simulink model "CodeGen"  (R2024b)
settings: Solver=FixedStepDiscrete  StartTime=0  StopTime=511  FixedStep=1/128  RelTol=1e-3
InitFcn:
  | load('ECG_Data_split.mat')
  | ecg_stream = timetable(testData','TimeStep',seconds(1/128));
  | classNames=["ARR","CHF","NSR"];
  | classNamesL=["arr","chf","nsr"];
  | path = ['CodeGen','/Subsystem/ECG Preprocessing/LSTM_Version/Resettable Subsystem/Stateful Classify1/'];
  | set_param(path,'InputDataFormats',"{'sequenceinput', 'CT'}");
undefined symbols (not defined in the file): gray
libraries: deeplib x2, dspfeatures x1, pil_lib x1
settings Model: Creator=The MathWorks, Inc.  LastModifiedBy=resjoehr
settings SolverCC: AlgebraicLoopSolver=TrustRegion
settings OptimizationCC: DefaultParameterBehavior=Inlined  EnhancedBackFolding=on  PassReuseOutputArgsAs=Individual arguments  ZeroExternalMemoryAtStartup=off  ZeroInternalMemoryAtStartup=off  InitFltsAndDblsToZero=on  MaxStackSize=200000  OptimizeBlockOrder=speed  DifferentSizesBufferReuse=on  OptimizationCustomize=off  EfficientTunableParamExpr=on
settings DebuggingCC: ParameterTunabilityLossMsg=error  UnconnectedInputMsg=warning  UnconnectedOutputMsg=warning  UnconnectedLineMsg=warning
settings HardwareCC: ProdBitPerLong=64  ProdLargestAtomicInteger=LongLong  ProdLargestAtomicFloat=Double  ProdLongLongMode=on  ProdHWDeviceType=ARM Compatible->ARM Cortex-A (64-bit)  TargetLongLongMode=on
settings ModelReferenceCC: EnableRefExpFcnMdlSchedulingChecks=on
settings SFSimCC: SimTargetLang=C++  SimGPUErrorChecks=on
settings RTWCC: Description=Embedded Coder  SystemTargetFile=ert.tlc  HardwareBoard=NVIDIA Jetson  TLCOptions="-aInlineSetEventsForThisBaseRateFcn=TLC_FALSE -aSuppressMultiTaskScheduler=TLC_FALSE  -aRateBasedStepFcn=0"  TemplateMakefile=ert_default_tmf  GenerateReport=on  LaunchReport=on  CreateSILPILBlock=PIL  TargetLang=C++  GenerateGPUCode=CUDA  GenerateCodeMetricsReport=on  GPUComputeCapability=3.5  DLArmComputeVersion=19.05
settings CodeAppCC: ForceParamTrailComments=on  IgnoreCustomStorageClasses=off  OperatorAnnotations=on  SimulinkDataObjDesc=on  SFDataObjDesc=on  InsertBlockDesc=on
settings ERTTargetCC: CodeInterfacePackaging=C++ class  SupportVariableSizeSignals=on  RootIOFormat=Structure reference  DynamicArrayContainerType=coder::array

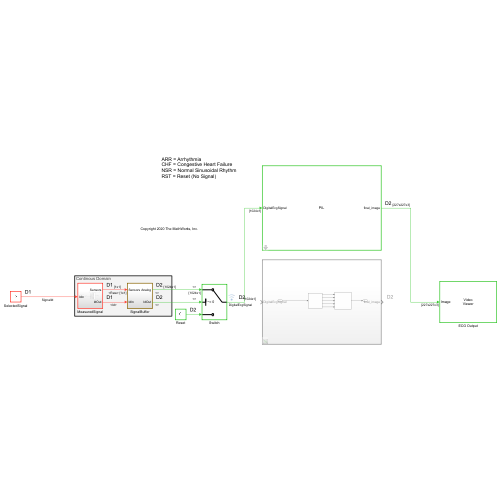
[thumbnail: Simulink's stored preview of the top-level diagram]
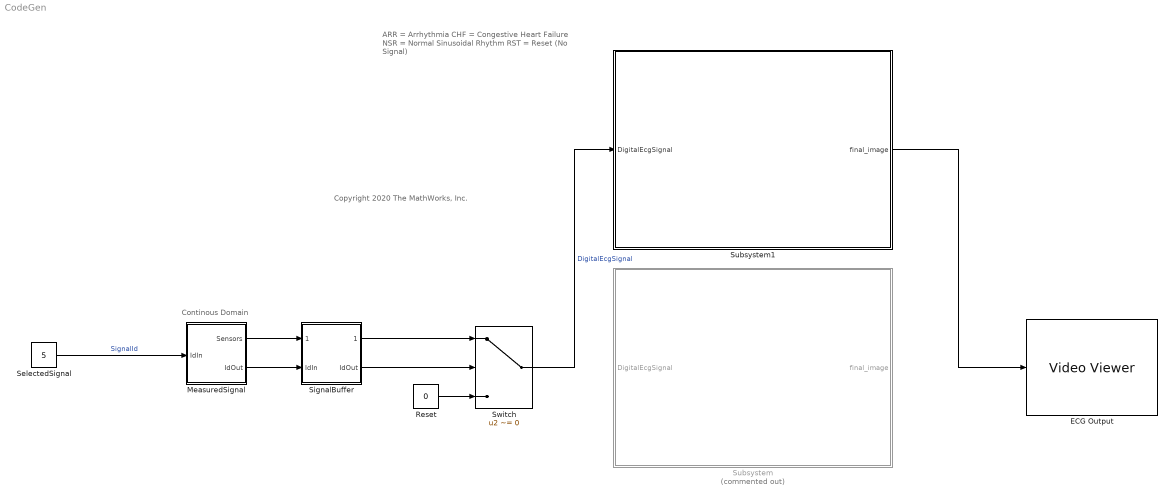
== system CodeGen ==
  note: Copyright 2020 The MathWorks, Inc.
  note: ARR = Arrhythmia
      | CHF = Congestive Heart Failure
      | NSR = Normal Sinusoidal Rhythm
      | RST = Reset (No Signal)
  note: Continous Domain
  ECG Output : VideoViewer  colormapValue=gray(256)  FigPos=[-1729 1066.66666666667 1030.66666666667 710]
  MeasuredSignal : Subsystem  VariantControl=testMixed
  Reset : Constant  Value=0  SampleTime=-1
  SelectedSignal : Constant  Value=5  SampleTime=-1
  SignalBuffer : Subsystem
  Subsystem : Subsystem  Commented=on  TreatAsAtomicUnit=on
  Subsystem1 : Subsystem  DialogController=pil_create_dialog  LoadFcn=|
      | try
      |    if ~strcmp(rtw.pil.getPILVersion, '24.2 (R2024b)_15')
      |       set_param(gcb, 'DialogController', '');
      |       set_param(gcb, 'DialogControllerArgs', '');
      |    end
      | catch e
      |       set_param(gcb, 'DialogController', '');
      |       set_param(gcb, 'DialogControllerArgs', '');
      | end
      mask help: PIL:pil:XILBlockMaskDesc
      mask Display: disp('PIL');
  Switch : Switch  Criteria=u2 ~= 0  OutDataTypeStr=Inherit: Inherit via back propagation  SaturateOnIntegerOverflow=off  InputSameDT=off
  wires:
  SignalBuffer/1(Analog) -> Switch/1
  SelectedSignal/1 -> MeasuredSignal/1(IdIn)  "SignalId"
  MeasuredSignal/1(Sensors) -> SignalBuffer/1(Sensors)
  SignalBuffer/2(IdOut) -> Switch/2
  MeasuredSignal/2(IdOut) -> SignalBuffer/2(IdIn)
  Reset/1 -> Switch/3
  Switch/1 -> Subsystem1/1(DigitalEcgSignal)  "DigitalEcgSignal"
  Subsystem1/1(final_image) -> ECG Output/1

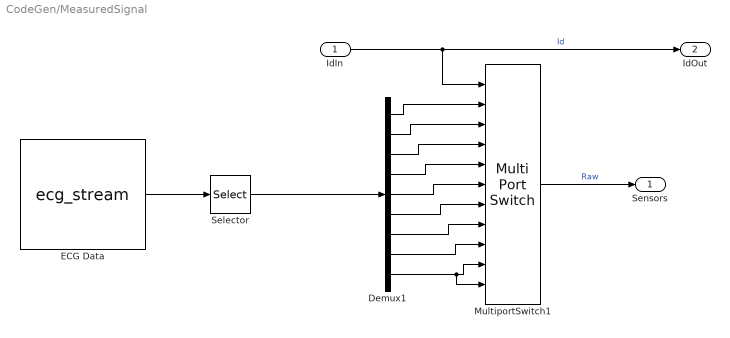
== system CodeGen/MeasuredSignal ==
  IdIn : Inport
  Demux1 : Demux  Outputs=9
  ECG Data : FromWorkspace  VariableName=ecg_stream  SampleTime=1/128
  MultiportSwitch1 : MultiPortSwitch  Inputs=9  DataPortForDefault=Additional data port  DiagnosticForDefault=None  SaturateOnIntegerOverflow=off  InputSameDT=off
  Selector : Selector  InputPortWidth=49  IndexOptions=Index vector (dialog)  Indices=[3 12 27 31 36 38 43 48 49]  OutputSizes=1
  Sensors : Outport
  IdOut : Outport  Port=2
  wires:
  IdIn/1 -> MultiportSwitch1/1, IdOut/1  "Id"
  Demux1/8 -> MultiportSwitch1/9
  Selector/1 -> Demux1/1
  Demux1/9 -> MultiportSwitch1/11, MultiportSwitch1/10
  Demux1/7 -> MultiportSwitch1/8
  Demux1/4 -> MultiportSwitch1/5
  Demux1/5 -> MultiportSwitch1/6
  MultiportSwitch1/1 -> Sensors/1  "Raw"
  ECG Data/1 -> Selector/1
  Demux1/6 -> MultiportSwitch1/7
  Demux1/1 -> MultiportSwitch1/2
  Demux1/3 -> MultiportSwitch1/4
  Demux1/2 -> MultiportSwitch1/3

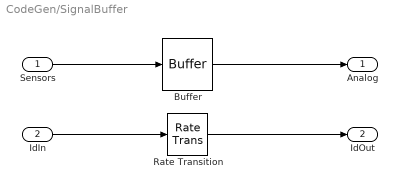
== system CodeGen/SignalBuffer ==
  Sensors : Inport
  IdIn : Inport  Port=2
  Buffer : Buffer  N=1024  V=512  OutputFrames=off
  Rate Transition : RateTransition  OutPortSampleTime=4
  Analog : Outport
  IdOut : Outport  Port=2
  wires:
  IdIn/1 -> Rate Transition/1
  Sensors/1 -> Buffer/1
  Buffer/1 -> Analog/1
  Rate Transition/1 -> IdOut/1

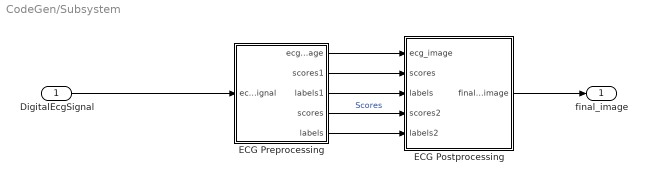
== system CodeGen/Subsystem ==
  DigitalEcgSignal : Inport
  ECG Postprocessing : MATLAB Function  TreatAsAtomicUnit=on
  ECG Preprocessing : Subsystem  TreatAsAtomicUnit=on
  final_image : Outport
  wires:
  ECG Preprocessing/4(scores) -> ECG Postprocessing/4(scores2)  "Scores"
  ECG Preprocessing/5(labels) -> ECG Postprocessing/5(labels2)
  ECG Preprocessing/1(ecg_image) -> ECG Postprocessing/1(ecg_image)
  DigitalEcgSignal/1 -> ECG Preprocessing/1(ecg_signal)
  ECG Postprocessing/1(final_image) -> final_image/1
  ECG Preprocessing/3(labels1) -> ECG Postprocessing/3(labels)
  ECG Preprocessing/2(scores1) -> ECG Postprocessing/2(scores)

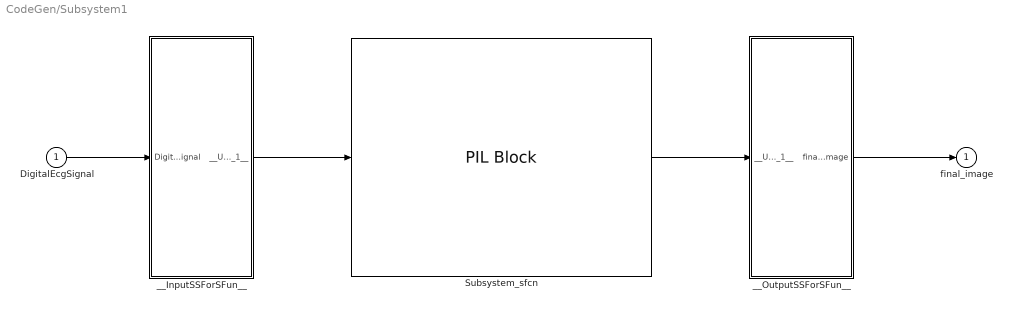
== system CodeGen/Subsystem1 ==
  DigitalEcgSignal : Inport
  Subsystem_sfcn : pil_lib/PIL Block  SimulationMode=PIL  IsTopModelPIL=off  CodeDir=Subsystem_ert_rtw  AnchorDir=C:\MATLAB\Content\D1_Artificial_Intelligence\M3_Workshops\AdaptedMaterial\AMLD_2025_final\Ch4_Deployment  ConfigName=NVIDIA Jetson  XrelIsTopModelCode=on  XrelIsReusable=off  XrelDWorkNames={}  XrelDWorkTypes={}  XrelModelArgVals={}  XrelOrderedParamNames={}  XRelNonFiniteStyle=NONFINITE_UNUSED
  __InputSSForSFun__ : Subsystem
  __OutputSSForSFun__ : Subsystem
  final_image : Outport
  wires:
  DigitalEcgSignal/1 -> __InputSSForSFun__/1(DigitalEcgSignal)
  __InputSSForSFun__/1(__UniqueOutportName__1__) -> Subsystem_sfcn/1
  Subsystem_sfcn/1 -> __OutputSSForSFun__/1(__UniqueInportName__1__)
  __OutputSSForSFun__/1(final_image) -> final_image/1

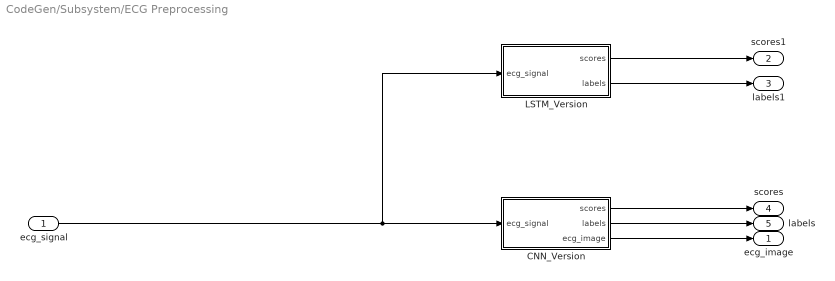
== system CodeGen/Subsystem/ECG Preprocessing ==
  ecg_signal : Inport
  CNN_Version : Subsystem  TreatAsAtomicUnit=on  VariantControl=false
      settings: RTWSystemCode=Nonreusable function
  LSTM_Version : Subsystem  TreatAsAtomicUnit=on  VariantControl=true
      settings: RTWSystemCode=Nonreusable function
  ecg_image : Outport
  scores1 : Outport  Port=2
  labels1 : Outport  Port=3
  scores : Outport  Port=4
  labels : Outport  Port=5
  wires:
  ecg_signal/1 -> LSTM_Version/1(ecg_signal), CNN_Version/1(ecg_signal)
  CNN_Version/3(ecg_image) -> ecg_image/1
  CNN_Version/2(labels) -> labels/1
  CNN_Version/1(scores) -> scores/1
  LSTM_Version/1(scores) -> scores1/1
  LSTM_Version/2(labels) -> labels1/1

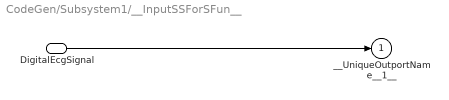
== system CodeGen/Subsystem1/__InputSSForSFun__ ==
  DigitalEcgSignal : Inport
  __UniqueOutportName__1__ : Outport
  wires:
  DigitalEcgSignal/1 -> __UniqueOutportName__1__/1

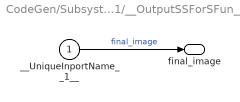
== system CodeGen/Subsystem1/__OutputSSForSFun__ ==
  __UniqueInportName__1__ : Inport
  final_image : Outport
  wires:
  __UniqueInportName__1__/1 -> final_image/1  "final_image"

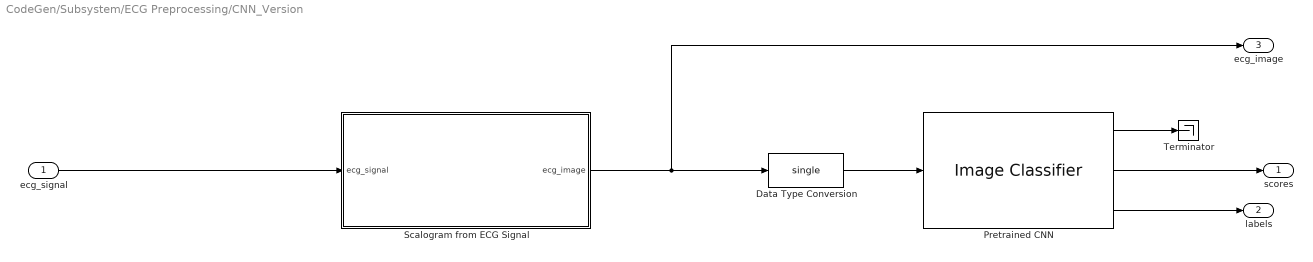
== system CodeGen/Subsystem/ECG Preprocessing/CNN_Version ==
  ecg_signal : Inport
  Data Type Conversion : DataTypeConversion  OutDataTypeStr=single  SaturateOnIntegerOverflow=off  RndMeth=Floor
  "Pretrained CNN " : deeplib/Image Classifier  Network=Network from MAT-file  NetworkFunction=squeezenet  NetworkFilePath=trained_GN.mat  NetworkClassesVariable=classNames  MiniBatchSize=128  ResizeInput=on  Classification=on  Predictions=on  ForceInterpretedSim=off  PredictMode=All probabilities and labels  K=5
  Scalogram from ECG Signal : MATLAB Function  TreatAsAtomicUnit=on
  Terminator : Terminator
  scores : Outport
  labels : Outport  Port=2
  ecg_image : Outport  Port=3
  wires:
  Data Type Conversion/1 -> "Pretrained CNN "/1
  Scalogram from ECG Signal/1(ecg_image) -> ecg_image/1, Data Type Conversion/1
  ecg_signal/1 -> Scalogram from ECG Signal/1(ecg_signal)
  "Pretrained CNN "/1 -> Terminator/1
  "Pretrained CNN "/2 -> scores/1
  "Pretrained CNN "/3 -> labels/1

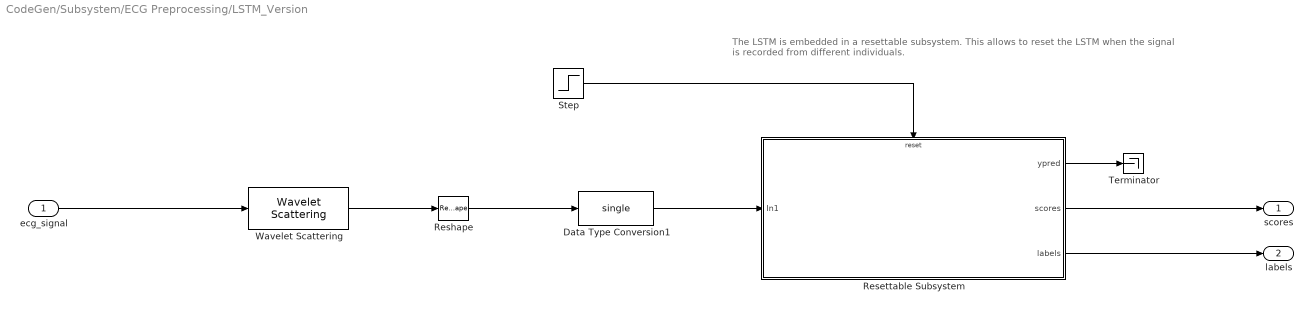
== system CodeGen/Subsystem/ECG Preprocessing/LSTM_Version ==
  note: The LSTM is embedded in a resettable subsystem. This allows to reset the LSTM when the signal is recorded from different individuals.
  ecg_signal : Inport
  Data Type Conversion1 : DataTypeConversion  OutDataTypeStr=single  SaturateOnIntegerOverflow=off  RndMeth=Floor
  Resettable Subsystem : Subsystem  TreatAsAtomicUnit=on
  Reshape : Reshape
  Step : Step  Time=0.1  SampleTime=4
  Terminator : Terminator
  Wavelet Scattering : dspfeatures/Wavelet Scattering  SignalLength=1024  OverlapLength=0  SpecifySampleRate=on  SampleRate=128  InvarianceScaleSamples=512  InvarianceScaleSeconds=4  QualityFactors=[8,1]  OptimizePath=off  OversamplingFactor=0  Boundary=periodic  IncludeZeroOrderCoeff=on  FeatureMatrixNormalization=none  FeatureMatrixTransform=none
  scores : Outport
  labels : Outport  Port=2
  wires:
  Reshape/1 -> Data Type Conversion1/1
  ecg_signal/1 -> Wavelet Scattering/1
  Wavelet Scattering/1 -> Reshape/1
  Data Type Conversion1/1 -> Resettable Subsystem/1(In1)
  Resettable Subsystem/2(scores) -> scores/1
  Resettable Subsystem/3(labels) -> labels/1
  Step/1 -> Resettable Subsystem/Reset
  Resettable Subsystem/1(ypred) -> Terminator/1

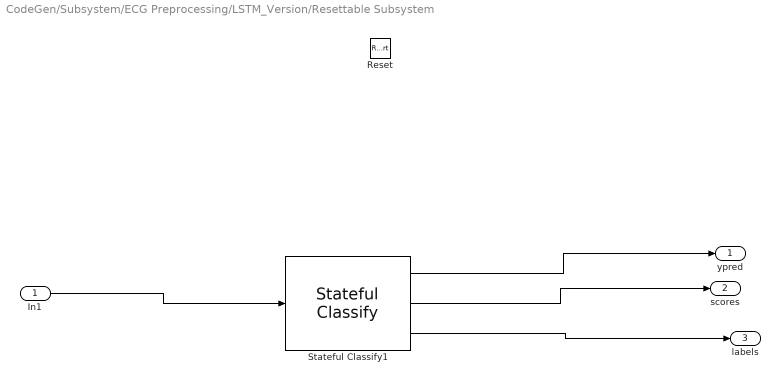
== system CodeGen/Subsystem/ECG Preprocessing/LSTM_Version/Resettable Subsystem ==
  In1 : Inport
  Reset : ResetPort  DisableCoverage=on
  Stateful Classify1 : deeplib/Stateful Classify  Network=Network from MAT-file  NetworkFunction=untitled  NetworkFilePath=LSTM.mat  NetworkClassesVariable=classNamesL  InputDataFormats={'sequenceinput', 'CT'}  SampleTime=-1  Classification=on  Predictions=on  ForceInterpretedSim=off  PredictMode=All probabilities and labels  K=5  LastKnownNetworkFilePath='LSTM.mat'  LastKnownNetworkTimeStamp=739655.493495370377786457538604736328125
  ypred : Outport
  scores : Outport  Port=2
  labels : Outport  Port=3
  wires:
  In1/1 -> Stateful Classify1/1
  Stateful Classify1/1 -> ypred/1
  Stateful Classify1/2 -> scores/1
  Stateful Classify1/3 -> labels/1

== matlab function CodeGen/Subsystem/ECG Postprocessing ==
  data: ecg_image input; final_image output; scores input; labels input; scores2 input; labels2 input
function final_image = ECGPostprocessing(ecg_image, scores, labels, scores2, labels2)
    
    final_image = label_prob_image2(ecg_image, scores, labels, scores2, labels2);

end

== matlab function CodeGen/Subsystem/ECG Preprocessing/CNN_Version/Scalogram from ECG Signal ==
  data: ecg_signal input; ecg_image output
function ecg_image  = ScalogramFromECG(ecg_signal)
    
    ecg_image = ecg_to_scalogram(ecg_signal);  

end
